simulink model "otonomvehicle"  (R2021b)
settings: Solver=VariableStepAuto  StartTime=0.0  StopTime=50  RelTol=1e-3
libraries: sim3dautolib x3, vrlib x2, simulink x2, sim3dlib x1, mpcadaslib x1, slpidlib x1
settings Model: Creator=serih  LastModifiedBy=serih

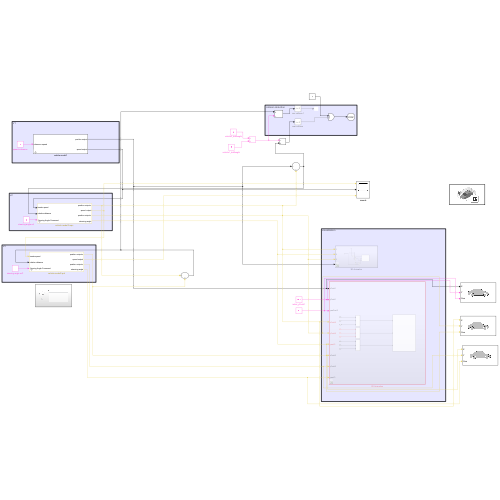
[thumbnail: Simulink's stored preview of the top-level diagram]
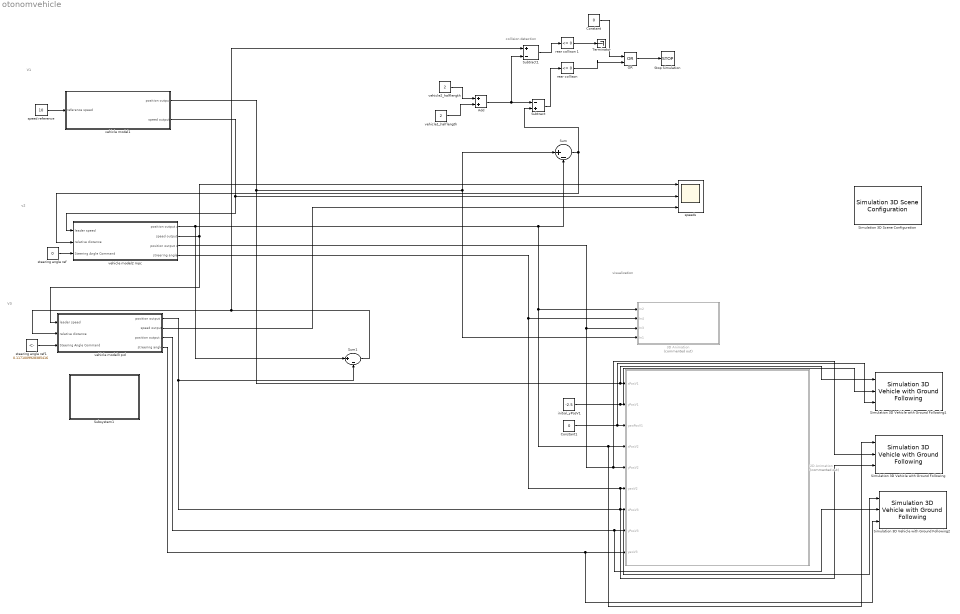
== system otonomvehicle ==
  note: V3
  note: v2
  note: V1
  note: visualization
  note: collision detection
  2D Animation : Subsystem  Commented=on  TreatAsAtomicUnit=on  SystemSampleTime=0.02
  3D Animation : Subsystem  Commented=on
  Add : Sum
  Constant : Constant  Value=0
  Constant1 : Constant  Value=0
  OR : Logic  Operator=OR  IconShape=distinctive  AllPortsSameDT=off  OutDataTypeStr=boolean
  Simulation 3D Scene Configuration : sim3dlib/Simulation 3D Scene Configuration  Priority=0  ProjectFormat_internal=Default Scenes  ProjectFormat=Default Scenes  SceneDesc=Straight road  ProjectName=C:\Program Files\MATLAB\R2021b\toolbox\shared\sim3d_projects\automotive_project\UE4\WindowsNoEditor\VehicleSimulation.exe  ScenePath=/Game/Maps/HwStrght  vehTagList={'Scene Origin';'SimulinkVehicle1';'SimulinkVehicle2';'SimulinkVehicle3'}  vehTag=SimulinkVehicle3  OpVisEn=off  Ts=0.1  EnableWindow=on  EnableWeather=off  SunAltitude=40.0  SunAzimuth=90  clouds=10  wind=1  fog=0  rain=0  sensorTag=MainCamera1  sensorId=1  sensorName=MainCamera1  mountLoc=Origin  offsetFlag=off  tmountOffset=[0, 0, 0]  rmountOffset=[0, 0, 0]  HorizontalResolution=1280  VerticalResolution=720  HorizontalFOV=60  mountPoint=[0 0 0]  mountOrientation=[0 0 0]  aMode=3  ID=1
      link override Simulation 3D Engine: SceneDesc=Straight road  EnableWeather=off  WeatherConfigParas=[40.0,90,10,0,0,1]
      settings: SourceProductBaseCode=AE,DR,UV,VE
  Simulation 3D Vehicle with Ground Following : sim3dautolib/Simulation 3D Vehicle with Ground Following  Priority=-1  PassVehMesh=Sport utility vehicle  PassVehMesh_Internal=Sport utility vehicle  MeshPath=/MathWorksSimulation/Vehicles/Muscle/Meshes/SK_MuscleCar.SK_MuscleCar  TrackWidth=1.9  WheelBase=3  WheelRadius=0.35  VehColor=Green  VehColor_Internal=Green  InitialPos=[20, 0, 0]  InitialRot=[0, 0, 0]  ActorName=SimulinkVehicle1  SampleTime=0.1  ActorType=SimulinkVehicle  ID=1  aMode=3  ActorTag=SimulinkVehicle1  CoordinateScheme=ISO  VehLightsControl=off  HeadlightColor=[ 1, 1, 1 ]  HighBeamIntensity=100000  LowBeamIntensity=60000  HighBeamConeAngle=70  LowBeamConeAngle=70  LeftHeadlightOrientation=[ 0, 0 ]  RightHeadlightOrientation=[ 0, 0 ]  BrakelightIntensity=500  ReverselightIntensity=500  SignallightIntensity=500  SignallightPeriod=1  SignalPulseWidth=50  TransformOutportEnabled=off
      settings: SourceProductBaseCode=AE,DR,UV,VE
  Simulation 3D Vehicle with Ground Following1 : sim3dautolib/Simulation 3D Vehicle with Ground Following  Priority=-1  PassVehMesh=Sedan  PassVehMesh_Internal=Sedan  MeshPath=/MathWorksSimulation/Vehicles/Muscle/Meshes/SK_MuscleCar.SK_MuscleCar  TrackWidth=1.9  WheelBase=3  WheelRadius=0.35  VehColor=Red  VehColor_Internal=Red  InitialPos=[40, 0, 0]  InitialRot=[0, 0, 0]  ActorName=SimulinkVehicle2  SampleTime=0.1  ActorType=SimulinkVehicle  ID=2  aMode=3  ActorTag=SimulinkVehicle2  CoordinateScheme=ISO  VehLightsControl=off  HeadlightColor=[ 1, 1, 1 ]  HighBeamIntensity=100000  LowBeamIntensity=60000  HighBeamConeAngle=70  LowBeamConeAngle=70  LeftHeadlightOrientation=[ 0, 0 ]  RightHeadlightOrientation=[ 0, 0 ]  BrakelightIntensity=500  ReverselightIntensity=500  SignallightIntensity=500  SignallightPeriod=1  SignalPulseWidth=50  TransformOutportEnabled=off
      settings: SourceProductBaseCode=AE,DR,UV,VE
  Simulation 3D Vehicle with Ground Following2 : sim3dautolib/Simulation 3D Vehicle with Ground Following  Priority=-1  PassVehMesh=Hatchback  PassVehMesh_Internal=Hatchback  MeshPath=/MathWorksSimulation/Vehicles/Muscle/Meshes/SK_MuscleCar.SK_MuscleCar  TrackWidth=1.9  WheelBase=3  WheelRadius=0.35  VehColor=Yellow  VehColor_Internal=Yellow  InitialPos=[0, 0, 0]  InitialRot=[0, 0, 0]  ActorName=SimulinkVehicle3  SampleTime=0.1  ActorType=SimulinkVehicle  ID=3  aMode=3  ActorTag=SimulinkVehicle3  CoordinateScheme=ISO  VehLightsControl=off  HeadlightColor=[ 1, 1, 1 ]  HighBeamIntensity=100000  LowBeamIntensity=60000  HighBeamConeAngle=70  LowBeamConeAngle=70  LeftHeadlightOrientation=[ 0, 0 ]  RightHeadlightOrientation=[ 0, 0 ]  BrakelightIntensity=500  ReverselightIntensity=500  SignallightIntensity=500  SignallightPeriod=1  SignalPulseWidth=50  TransformOutportEnabled=off
      settings: SourceProductBaseCode=AE,DR,UV,VE
  Stop Simulation : Stop
  Subsystem1 : Subsystem
  Subtract : Sum  Inputs=-+
  Subtract1 : Sum  Inputs=+-
  Sum : Sum  Inputs=|+-
  Sum1 : Sum  Inputs=|+-
  Terminator : Terminator
  initial_yPosV1 : Constant  Value=-2.5
  "rear collison " : simulink/Logic and Bit Operations/Compare To Constant  relop=<=  const=0  OutDataTypeStr=boolean
  rear collison 1 : simulink/Logic and Bit Operations/Compare To Constant  relop=<=  const=0  OutDataTypeStr=boolean
  speed reference : Constant  Value=10
  speeds : Scope  NumInputPorts=3
  steering angle ref : Constant  Value=0  VectorParams1D=off
  steering angle ref1 : Constant  Value=0.1171009928385416  VectorParams1D=off
  vehicle model1 : Subsystem  mask{pos=30, speed=20}
      mask prompts: pos "initial position"; speed "initial speed"
      mask TypeOptions pos: initial position/Value
      mask TypeOptions speed: initial speed/Value
  "vehicle model2 mpc " : Subsystem  mask{pos=20, speed=15}
      mask prompts: pos "initial position"; speed "initial speed"
      mask TypeOptions pos: initial position z/Value
      mask TypeOptions speed: initial speed/Value
  vehicle model3 pıd : Subsystem  mask{pos=0, speed=20}
      mask prompts: pos "initial position"; speed "initial speed"
      mask TypeOptions pos: initial position z/Value
      mask TypeOptions speed: initial speed/Value
  vehicle1_halflength : Constant  Value=2
  vehicle2_halflength : Constant  Value=2
  wires:
  speed reference/1 -> vehicle model1/1(reference speed)
  vehicle model1/1(position output) -> Simulation 3D Vehicle with Ground Following1/1, 2D Animation/1(xPosV1), 3D Animation/4(In1), Sum/1
  "vehicle model2 mpc "/1(position output z) -> Sum1/1, Sum/2, 3D Animation/1(In2), Simulation 3D Vehicle with Ground Following/1, 2D Animation/4(xPosV2)
  vehicle model1/2(speed output) -> speeds/2, "vehicle model2 mpc "/1(leader speed)
  Sum/1 -> Subtract/2, "vehicle model2 mpc "/2(relative distance)
  steering angle ref/1 -> "vehicle model2 mpc "/3(Steering Angle Command)
  "vehicle model2 mpc "/3(position output x) -> Simulation 3D Vehicle with Ground Following/2, 2D Animation/5(yPosV2), 3D Animation/3(In3)
  "vehicle model2 mpc "/4(streering angle) -> Simulation 3D Vehicle with Ground Following/3, 2D Animation/6(yawV2), 3D Animation/2(In4)
  Constant1/1 -> 2D Animation/3(yawPosV1), Simulation 3D Vehicle with Ground Following1/3
  initial_yPosV1/1 -> Simulation 3D Vehicle with Ground Following1/2, 2D Animation/2(yPosV1)
  vehicle2_halflength/1 -> Add/1
  vehicle1_halflength/1 -> Add/2
  Add/1 -> Subtract1/2, Subtract/1
  Subtract/1 -> "rear collison "/1
  Subtract1/1 -> rear collison 1/1
  OR/1 -> Stop Simulation/1
  "rear collison "/1 -> OR/2
  "vehicle model2 mpc "/2(speed output) -> vehicle model3 pıd/1(leader speed), speeds/1
  vehicle model3 pıd/1(position output z) -> Simulation 3D Vehicle with Ground Following2/1, 2D Animation/7(xPosV3), Sum1/2
  Sum1/1 -> vehicle model3 pıd/2(relative distance), Subtract1/1
  steering angle ref1/1 -> vehicle model3 pıd/3(Steering Angle Command)
  vehicle model3 pıd/2(speed output) -> speeds/3
  vehicle model3 pıd/4(streering angle) -> Simulation 3D Vehicle with Ground Following2/3, 2D Animation/9(yawV3)
  vehicle model3 pıd/3(position output x) -> 2D Animation/8(yPosV3), Simulation 3D Vehicle with Ground Following2/2
  rear collison 1/1 -> Terminator/1
  Constant/1 -> OR/1

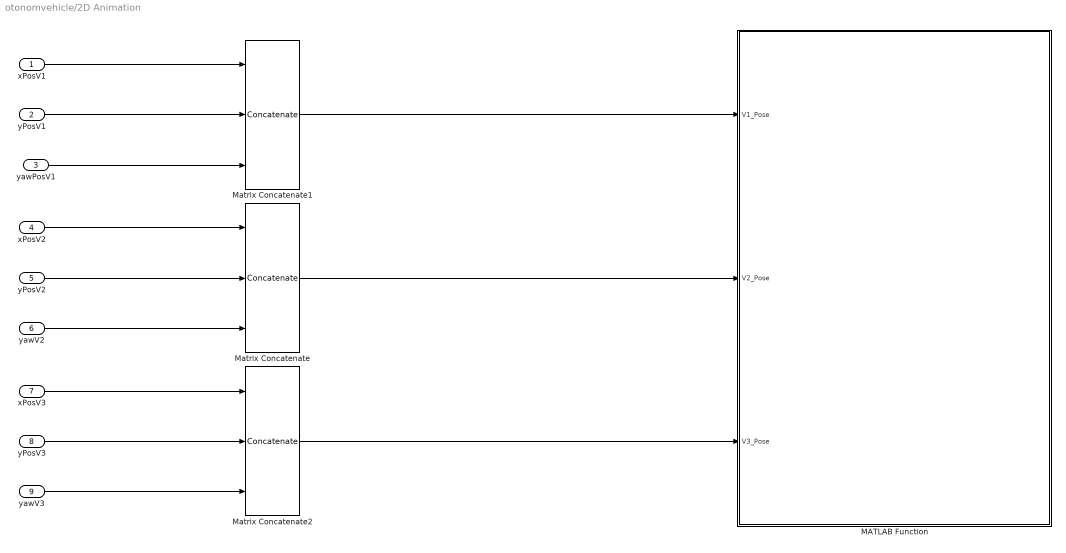
== system otonomvehicle/2D Animation ==
  xPosV1 : Inport
  yPosV1 : Inport  Port=2
  yawPosV1 : Inport  Port=3
  xPosV2 : Inport  Port=4
  yPosV2 : Inport  Port=5
  yawV2 : Inport  Port=6
  xPosV3 : Inport  Port=7
  yPosV3 : Inport  Port=8
  yawV3 : Inport  Port=9
  MATLAB Function : MATLAB Function  TreatAsAtomicUnit=on
      mask init:
      | close all;
      | figure('units','normalized','outerposition',[0 0 1 1 ]);
      | grid on
      | axis equal
      | hold on
  Matrix Concatenate : Concatenate  NumInputs=3  ConcatenateDimension=2
  Matrix Concatenate1 : Concatenate  NumInputs=3  ConcatenateDimension=2
  Matrix Concatenate2 : Concatenate  NumInputs=3  ConcatenateDimension=2
  wires:
  xPosV2/1 -> Matrix Concatenate/1
  yPosV2/1 -> Matrix Concatenate/2
  yawV2/1 -> Matrix Concatenate/3
  Matrix Concatenate/1 -> MATLAB Function/2(V2_Pose)
  Matrix Concatenate1/1 -> MATLAB Function/1(V1_Pose)
  xPosV1/1 -> Matrix Concatenate1/1
  yPosV1/1 -> Matrix Concatenate1/2
  yawPosV1/1 -> Matrix Concatenate1/3
  xPosV3/1 -> Matrix Concatenate2/1
  yPosV3/1 -> Matrix Concatenate2/2
  yawV3/1 -> Matrix Concatenate2/3
  Matrix Concatenate2/1 -> MATLAB Function/3(V3_Pose)

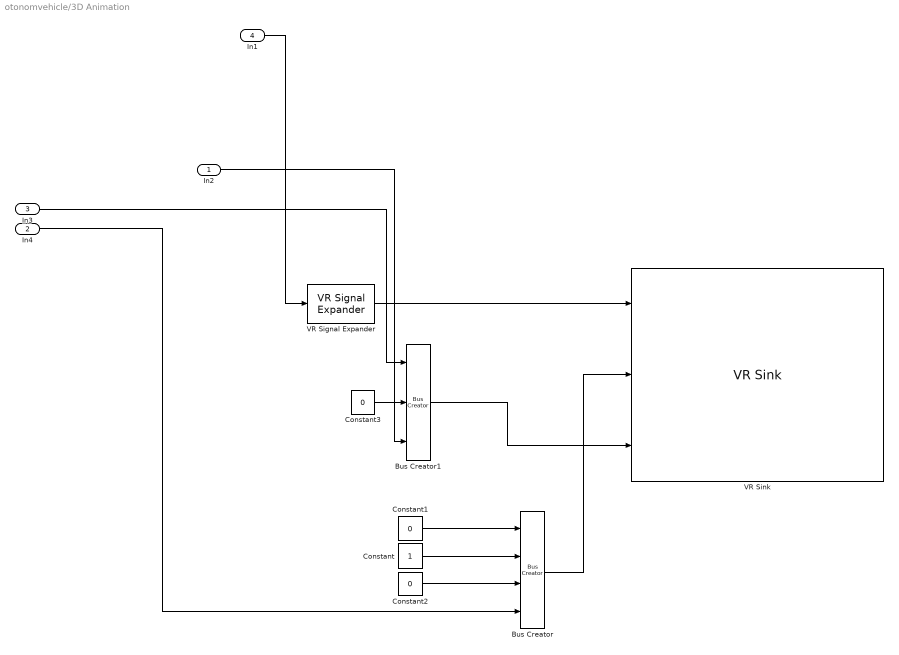
== system otonomvehicle/3D Animation ==
  In2 : Inport
  In4 : Inport  Port=2
  In3 : Inport  Port=3
  In1 : Inport  Port=4
  Bus Creator : BusCreator  Inputs=4
  Bus Creator1 : BusCreator  Inputs=3
  Constant : Constant
  Constant1 : Constant  Value=0
  Constant2 : Constant  Value=0
  Constant3 : Constant  Value=0
  VR Signal Expander : vrlib/VR Signal Expander  outwidth=3  outidx=[3]
  VR Sink : vrlib/VR Sink  InstantiateOnLoad=on  SampleTime=0.02  ViewEnable=on  RemoteChange=off  RemoteView=off  FieldsWritten=Car_Red.translation.3.1.1.double#Car_Blue.rotation.4.1.1.double#Car_Blue.translation.3.1.1.double  WorldFileName=OneDrive\Masaüstü\PlatoonWorld.WRL  AutoView=off  VideoDimensions=[]  AllowVariableSize=off
  wires:
  Constant1/1 -> Bus Creator/1
  VR Signal Expander/1 -> VR Sink/1
  In1/1 -> VR Signal Expander/1
  Constant2/1 -> Bus Creator/3
  Bus Creator/1 -> VR Sink/2
  Constant3/1 -> Bus Creator1/2
  Constant/1 -> Bus Creator/2
  Bus Creator1/1 -> VR Sink/3
  In3/1 -> Bus Creator1/1
  In4/1 -> Bus Creator/4
  In2/1 -> Bus Creator1/3

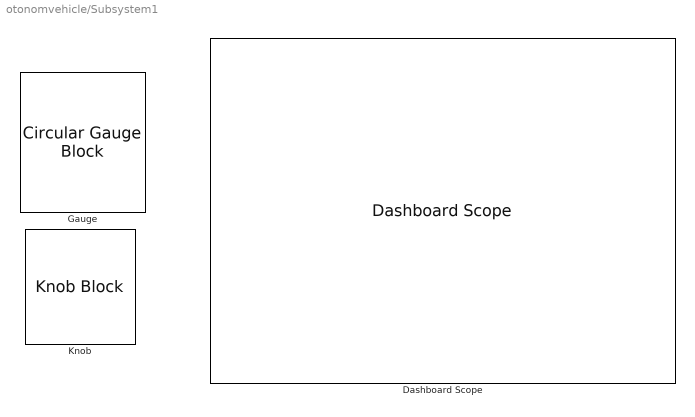
== system otonomvehicle/Subsystem1 ==
  Dashboard Scope : DashboardScope
  Gauge : CircularGaugeBlock
  Knob : KnobBlock  ScaleMin=-0.2  ScaleMax=0.2

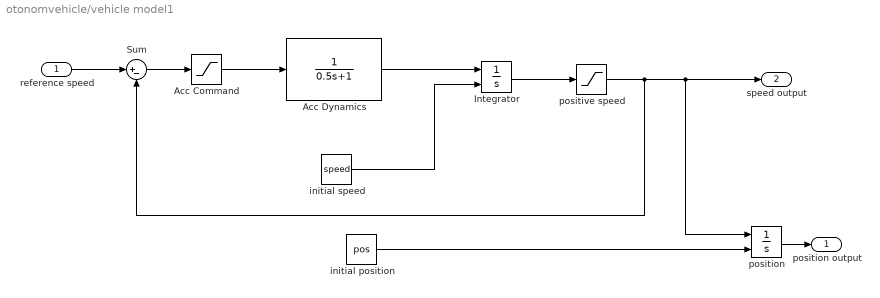
== system otonomvehicle/vehicle model1 ==
  reference speed : Inport
  Acc Command : Saturate  UpperLimit=2  LowerLimit=-3
  Acc Dynamics : TransferFcn  Denominator=[0.5 1]
  Integrator : Integrator  InitialConditionSource=external
  Sum : Sum  Inputs=|+-
  initial position : Constant  Value=pos
  initial speed : Constant  Value=speed
  position : Integrator  InitialConditionSource=external
  positive speed : Saturate  UpperLimit=inf  LowerLimit=0
  position output : Outport
  speed output : Outport  Port=2
  wires:
  Sum/1 -> Acc Command/1
  positive speed/1 -> speed output/1, position/1, Sum/2
  initial speed/1 -> Integrator/2
  initial position/1 -> position/2
  Acc Command/1 -> Acc Dynamics/1
  reference speed/1 -> Sum/1
  Acc Dynamics/1 -> Integrator/1
  Integrator/1 -> positive speed/1
  position/1 -> position output/1

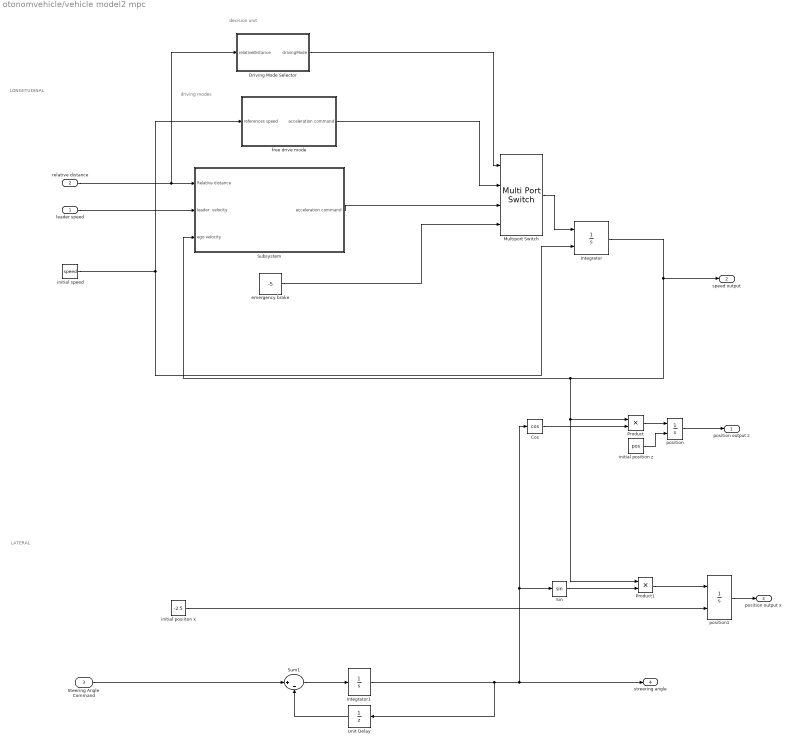
== system otonomvehicle/vehicle model2 mpc  ==
  note: decision unit
  note: driving modes
  note: LATERAL
  note: LONGIITUDINAL
  leader speed : Inport
  relative distance : Inport  Port=2
  Steering Angle Command : Inport  Port=3
  Cos : Trigonometry  Operator=cos
  Driving Mode Selector : Stateflow chart  TreatAsAtomicUnit=on
  Integrator : Integrator  InitialConditionSource=external  LimitOutput=on  LowerSaturationLimit=0
  Integrator1 : Integrator
  Multiport Switch : MultiPortSwitch
  Product : Product
  Product1 : Product
  Sin : Trigonometry
  Subsystem : Subsystem
  Sum1 : Sum  Inputs=|+-
  Unit Delay : UnitDelay  SampleTime=-1  HasFrameUpgradeWarning=on
  emergency brake : Constant  Value=-5
  free drive mode : Subsystem
  initial posiiton x : Constant  Value=-2.5
  initial position z : Constant  Value=pos
  initial speed : Constant  Value=speed
  position : Integrator  InitialConditionSource=external
  position1 : Integrator  InitialConditionSource=external
  position output z : Outport
  speed output : Outport  Port=2
  position output x : Outport  Port=3
  streering angle : Outport  Port=4
  wires:
  initial speed/1 -> Integrator/2, free drive mode/1(references speed)
  initial position z/1 -> position/2
  position/1 -> position output z/1
  Integrator/1 -> Subsystem/3("ego velocity "), Product1/1, Product/1, speed output/1
  Steering Angle Command/1 -> Sum1/1
  Sum1/1 -> Integrator1/1
  Integrator1/1 -> Unit Delay/1, streering angle/1, Cos/1, Sin/1
  Unit Delay/1 -> Sum1/2
  initial posiiton x/1 -> position1/2
  Cos/1 -> Product/2
  Product/1 -> position/1
  Sin/1 -> Product1/2
  Product1/1 -> position1/1
  position1/1 -> position output x/1
  relative distance/1 -> Driving Mode Selector/1(relativeDistance), Subsystem/1(Relative distance)
  leader speed/1 -> Subsystem/2("leader  velocity ")
  Multiport Switch/1 -> Integrator/1
  emergency brake/1 -> Multiport Switch/4
  Subsystem/1("acceleration command ") -> Multiport Switch/3
  free drive mode/1(acceleration command) -> Multiport Switch/2
  Driving Mode Selector/1(drivingMode) -> Multiport Switch/1

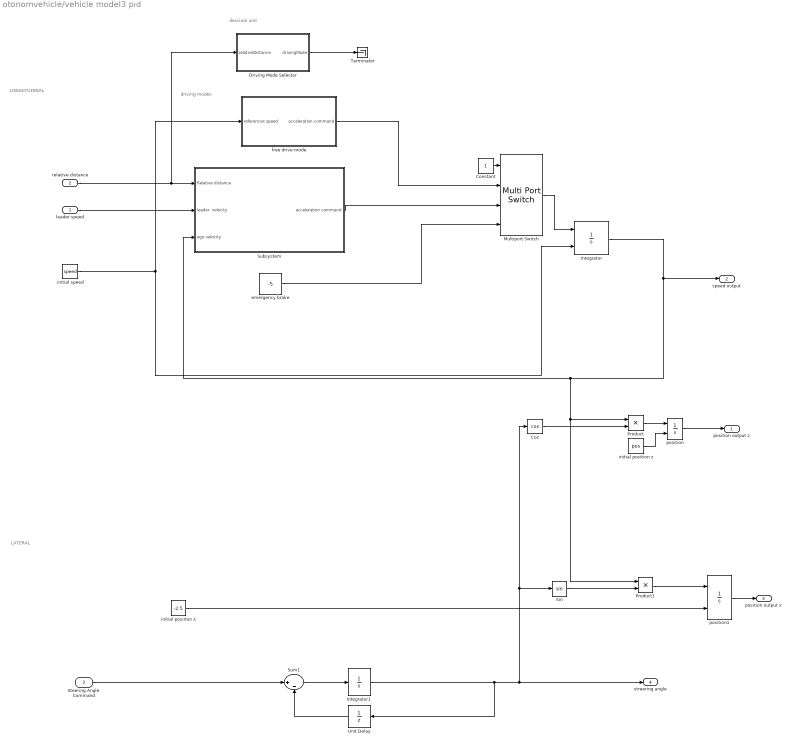
== system otonomvehicle/vehicle model3 pıd ==
  note: decision unit
  note: driving modes
  note: LATERAL
  note: LONGIITUDINAL
  leader speed : Inport
  relative distance : Inport  Port=2
  Steering Angle Command : Inport  Port=3
  Constant : Constant
  Cos : Trigonometry  Operator=cos
  Driving Mode Selector : Stateflow chart  TreatAsAtomicUnit=on
  Integrator : Integrator  InitialConditionSource=external  LimitOutput=on
  Integrator1 : Integrator
  Multiport Switch : MultiPortSwitch
  Product : Product
  Product1 : Product
  Sin : Trigonometry
  Subsystem : Subsystem
  Sum1 : Sum  Inputs=|+-
  Terminator : Terminator
  Unit Delay : UnitDelay  SampleTime=-1  HasFrameUpgradeWarning=on
  emergency brake : Constant  Value=-5
  free drive mode : Subsystem
  initial posiiton x : Constant  Value=-2.5
  initial position z : Constant  Value=pos
  initial speed : Constant  Value=speed
  position : Integrator  InitialConditionSource=external
  position1 : Integrator  InitialConditionSource=external
  position output z : Outport
  speed output : Outport  Port=2
  position output x : Outport  Port=3
  streering angle : Outport  Port=4
  wires:
  initial speed/1 -> Integrator/2, free drive mode/1(references speed)
  initial position z/1 -> position/2
  position/1 -> position output z/1
  Integrator/1 -> Subsystem/3("ego velocity "), Product1/1, Product/1, speed output/1
  Steering Angle Command/1 -> Sum1/1
  Sum1/1 -> Integrator1/1
  Integrator1/1 -> Unit Delay/1, streering angle/1, Cos/1, Sin/1
  Unit Delay/1 -> Sum1/2
  initial posiiton x/1 -> position1/2
  Cos/1 -> Product/2
  Product/1 -> position/1
  Sin/1 -> Product1/2
  Product1/1 -> position1/1
  position1/1 -> position output x/1
  relative distance/1 -> Driving Mode Selector/1(relativeDistance), Subsystem/1(Relative distance)
  leader speed/1 -> Subsystem/2("leader  velocity ")
  Multiport Switch/1 -> Integrator/1
  emergency brake/1 -> Multiport Switch/4
  Subsystem/1("acceleration command ") -> Multiport Switch/3
  free drive mode/1(acceleration command) -> Multiport Switch/2
  Driving Mode Selector/1(drivingMode) -> Terminator/1
  Constant/1 -> Multiport Switch/1

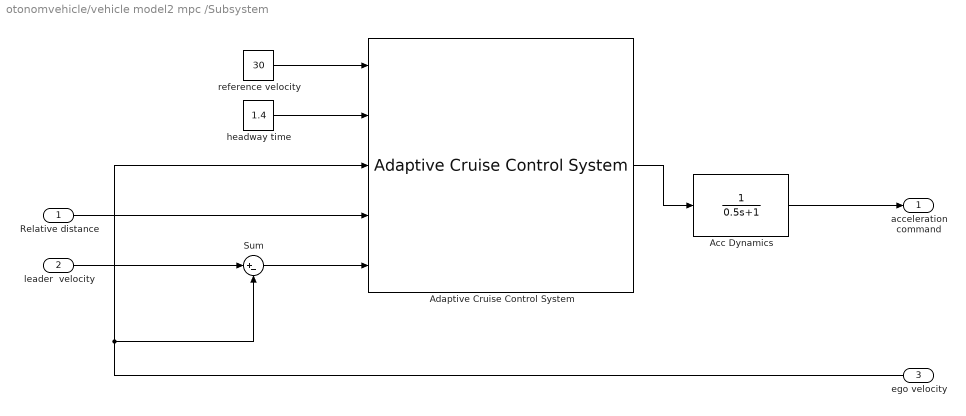
== system otonomvehicle/vehicle model2 mpc /Subsystem ==
  Relative distance : Inport
  "leader  velocity " : Inport  Port=2
  "ego velocity " : Inport  Port=3
  Acc Dynamics : TransferFcn  Denominator=[0.5 1]
  Adaptive Cruise Control System : mpcadaslib/Adaptive Cruise Control System  EgoModel=tf(1,[0.5,1,0])  InitialEgoVelocity=30  DefaultSpacing=10  MaxVelocity=50  MinAcceleration=-3  amin_ext=off  MaxAcceleration=2  amax_ext=off  Ts=0.5  PredictionHorizon=200  ControllerBehavior=0.590  suboptimal=off  maxiter=10  datatypeopt=double  optmode=off  trackmode=off
  Sum : Sum  Inputs=|+-
  headway time : Constant  Value=1.4
  reference velocity : Constant  Value=30
  "acceleration command " : Outport
  wires:
  Sum/1 -> Adaptive Cruise Control System/5
  headway time/1 -> Adaptive Cruise Control System/2
  Adaptive Cruise Control System/1 -> Acc Dynamics/1
  Acc Dynamics/1 -> "acceleration command "/1
  "leader  velocity "/1 -> Sum/1
  "ego velocity "/1 -> Sum/2, Adaptive Cruise Control System/3
  reference velocity/1 -> Adaptive Cruise Control System/1
  Relative distance/1 -> Adaptive Cruise Control System/4

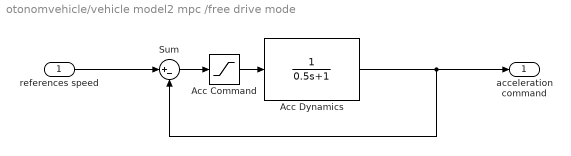
== system otonomvehicle/vehicle model2 mpc /free drive mode ==
  references speed : Inport
  Acc Command : Saturate  UpperLimit=2  LowerLimit=-3
  Acc Dynamics : TransferFcn  Denominator=[0.5 1]
  Sum : Sum  Inputs=|+-
  acceleration command : Outport
  wires:
  Sum/1 -> Acc Command/1
  references speed/1 -> Sum/1
  Acc Dynamics/1 -> Sum/2, acceleration command/1
  Acc Command/1 -> Acc Dynamics/1

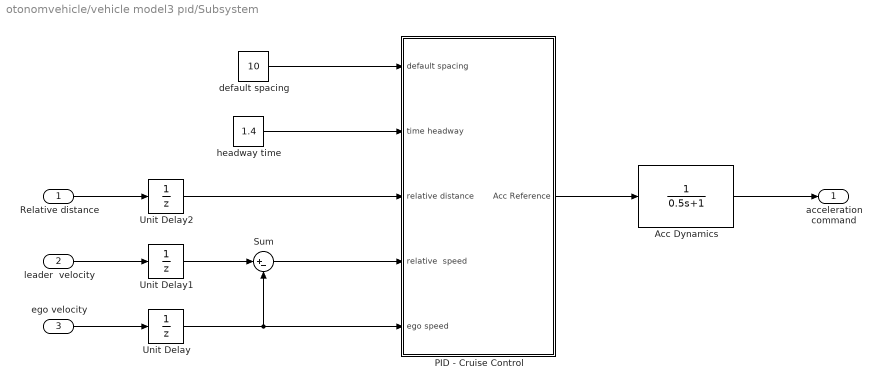
== system otonomvehicle/vehicle model3 pıd/Subsystem ==
  Relative distance : Inport
  "leader  velocity " : Inport  Port=2
  "ego velocity " : Inport  Port=3
  " default spacing" : Constant  Value=10
  Acc Dynamics : TransferFcn  Denominator=[0.5 1]
  PID - Cruise Control : Subsystem
  Sum : Sum  Inputs=|+-
  Unit Delay : UnitDelay  SampleTime=-1  HasFrameUpgradeWarning=on
  Unit Delay1 : UnitDelay  SampleTime=-1  HasFrameUpgradeWarning=on
  Unit Delay2 : UnitDelay  SampleTime=-1  HasFrameUpgradeWarning=on
  headway time : Constant  Value=1.4
  "acceleration command " : Outport
  wires:
  Sum/1 -> PID - Cruise Control/4(relative  speed)
  headway time/1 -> PID - Cruise Control/2(time headway)
  PID - Cruise Control/1(Acc Reference) -> Acc Dynamics/1
  Acc Dynamics/1 -> "acceleration command "/1
  Relative distance/1 -> Unit Delay2/1
  " default spacing"/1 -> PID - Cruise Control/1(default spacing)
  "ego velocity "/1 -> Unit Delay/1
  Unit Delay/1 -> Sum/2, PID - Cruise Control/5(ego speed)
  "leader  velocity "/1 -> Unit Delay1/1
  Unit Delay1/1 -> Sum/1
  Unit Delay2/1 -> PID - Cruise Control/3(relative distance)

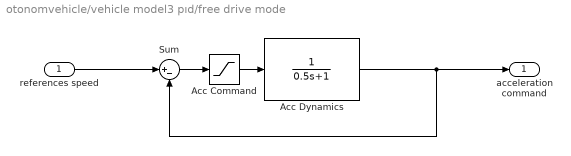
== system otonomvehicle/vehicle model3 pıd/free drive mode ==
  references speed : Inport
  Acc Command : Saturate  UpperLimit=2  LowerLimit=-3
  Acc Dynamics : TransferFcn  Denominator=[0.5 1]
  Sum : Sum  Inputs=|+-
  acceleration command : Outport
  wires:
  Sum/1 -> Acc Command/1
  references speed/1 -> Sum/1
  Acc Dynamics/1 -> Sum/2, acceleration command/1
  Acc Command/1 -> Acc Dynamics/1

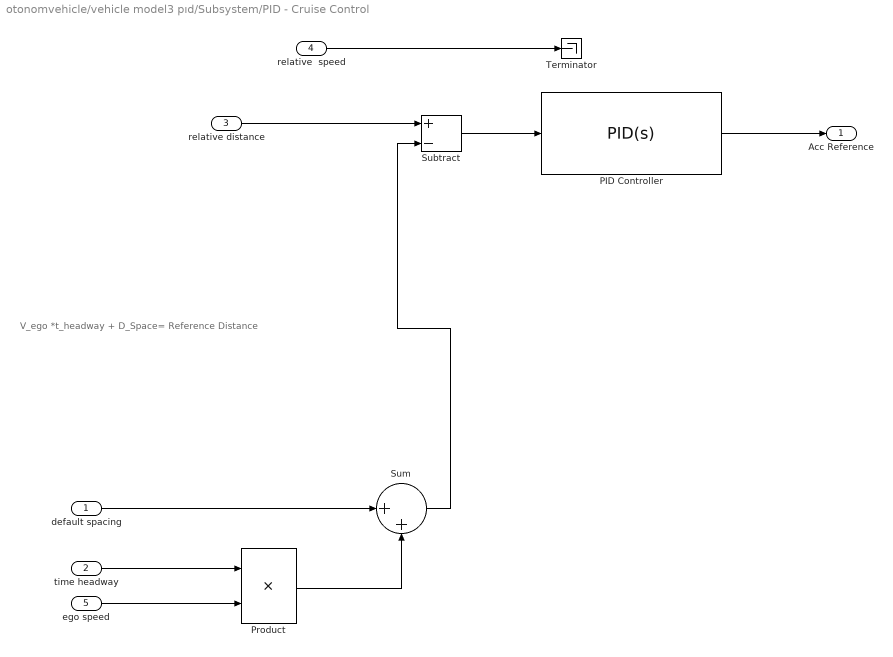
== system otonomvehicle/vehicle model3 pıd/Subsystem/PID - Cruise Control ==
  note: V_ego *t_headway + D_Space= Reference Distance
  default spacing : Inport
  time headway : Inport  Port=2
  relative distance : Inport  Port=3
  relative  speed : Inport  Port=4
  ego speed : Inport  Port=5
  PID Controller : slpidlib/PID Controller  Controller=PID  Form=Parallel  TimeDomain=Continuous-time  UseExternalTs=off  SampleTime=-1  IntegratorMethod=Forward Euler  FilterMethod=Forward Euler  ControllerParametersSource=internal  P=2  I=0.04  D=2.1  UseFilter=on  N=230  TunerSelectOption=Transfer Function Based (PID Tuner App)  InitialConditionSource=internal  InitialConditionForIntegrator=0  InitialConditionForFilter=0  DifferentiatorICPrevScaledInput=0  ExternalReset=none  TrackingMode=off  Kt=1  LimitOutput=on  SatLimitsSource=internal  UpperSaturationLimit=2  LowerSaturationLimit=-3  LinearizeAsGain=on  AntiWindupMode=clamping  Kb=1  POutMin=[]  POutMax=[]  IOutMin=[]  IOutMax=[]  DOutMin=[]  DOutMax=[]  NOutMin=[]  NOutMax=[]  SumOutMin=[]  SumOutMax=[]  SaturationOutMin=[]  SaturationOutMax=[]  PParamMin=[]  PParamMax=[]  IParamMin=[]  IParamMax=[]  DParamMin=[]  DParamMax=[]  NParamMin=[]  NParamMax=[]  KbParamMin=[]  KbParamMax=[]  KtParamMin=[]  KtParamMax=[]  KbOutMin=[]  KbOutMax=[]  KtOutMin=[]  KtOutMax=[]  IntegratorOutMin=[]  IntegratorOutMax=[]  FilterOutMin=[]  FilterOutMax=[]  SumI1OutMin=[]  SumI1OutMax=[]  SumI2OutMin=[]  SumI2OutMax=[]  SumI3OutMin=[]  SumI3OutMax=[]  SumI4OutMin=[]  SumI4OutMax=[]  SumDOutMin=[]  SumDOutMax=[]  DifferentiatorOutMin=[]  DifferentiatorOutMax=[]  FilterDiffOutCoefMin=[]  FilterDiffOutCoefMax=[]  ReciprocalOutMin=[]  ReciprocalOutMax=[]  SumDenOutMin=[]  SumDenOutMax=[]  SumNumOutMin=[]  SumNumOutMax=[]  DivideOutMin=[]  DivideOutMax=[]  UdiffTsProdOutMin=[]  UdiffTsProdOutMax=[]  NTsProdOutMin=[]  NTsProdOutMax=[]  UintegralTsProdOutMin=[]  UintegralTsProdOutMax=[]  UngainTsProdOutMin=[]  UngainTsProdOutMax=[]  IntegratorContinuousStateAttributes=''  IntegratorStateMustResolveToSignalObject=off  IntegratorRTWStateStorageClass=Auto  FilterContinuousStateAttributes=''  FilterStateMustResolveToSignalObject=off  FilterRTWStateStorageClass=Auto  ParallelPVariant=InternalParameters  IdealPVariant=Disabled  IVariant=InternalParameters  DVariant=InternalParameters  IntegratorVariant=Continuous  SatVariant=Enabled  AWVariant=ContClampingParallel  PCopyVariant=Disabled  TRVariant=Disabled  FdbkBlocksVariant=Forward  IdealPFdbkVariant=Disabled  SatFdbkVariant=Disabled  DerivativeFilterVariant=ContFilter  NVariant=InternalParameters  NCopyVariant=Disabled  FilterICVariant=InternalICsFilter  IntegratorICVariant=InternalICs  ExternalResetVariant=Disabled  TRSumVariant=Passthrough  SumFdbkVariant=Disabled  SumVariant=Sum_PID  TsampFilterVariant=InternalTs  TsampNgainVariant=Passthrough  TsampIntegralVariant=Passthrough  ExternalSaturationOutDataTypeStr=Inherit: Same as second input
  Product : Product
  Subtract : Sum  Inputs=+-
  Sum : Sum  Inputs=|++
  Terminator : Terminator
  Acc Reference : Outport
  wires:
  ego speed/1 -> Product/2
  time headway/1 -> Product/1
  Product/1 -> Sum/2
  default spacing/1 -> Sum/1
  Sum/1 -> Subtract/2
  relative distance/1 -> Subtract/1
  Subtract/1 -> PID Controller/1
  PID Controller/1 -> Acc Reference/1
  relative  speed/1 -> Terminator/1

== stateflow chart otonomvehicle/vehicle model3 pıd/Driving Mode Selector ==
  state FreeDrive
    entry:
    drivingMode=1;
  state VehicleFollowing
    entry:
    drivingMode=2;
  state EmergencyBrake
    entry:
    drivingMode=3;
  (default) -> FreeDrive
  VehicleFollowing -> FreeDrive [order 1] : [relativeDistance>50]
  FreeDrive -> VehicleFollowing : [relativeDistance <=40]
  EmergencyBrake -> FreeDrive [order 1] : [relativeDistance<=10]
  VehicleFollowing -> EmergencyBrake [order 2] : [relativeDistance<=10]
  EmergencyBrake -> VehicleFollowing [order 2] : [relativeDistance>15]
  data: relativeDistance input; drivingMode output

== matlab function otonomvehicle/2D Animation/MATLAB Function ==
  data: V1_Pose input; V2_Pose input; V3_Pose input
function plotVehicle(V1_Pose,V2_Pose,V3_Pose)
%%clear previous vehicle 
cla
%% vehicle-1 pose
x1=V1_Pose(1);
y1=V1_Pose(2);
yaw1=V1_Pose(3);
centerP=[x1;y1];

V1_HalfLength=2; %length 4 meters
V1_HalfWidth=1; %width 2 meters 

%creating a rectangle
p1=[V1_HalfLength; V1_HalfWidth];
p2=[V1_HalfLength; -V1_HalfWidth];
p3=[-V1_HalfLength; -V1_HalfWidth];
p4=[-V1_HalfLength; V1_HalfWidth];

%rotation matrix
Rmatrix=[cos(yaw1) -sin(yaw1);  sin(yaw1) cos(yaw1)];

%rotated points
p1r= centerP + Rmatrix*p1;
p2r= centerP + Rmatrix*p2;
p3r= centerP + Rmatrix*p3;
p4r= centerP + Rmatrix*p4;

%connecting points
Hitbox_V1= [p1r p2r p3r p4r p1r];

cornersV1_x= transpose(Hitbox_V1(1,:));
cornersV1_y= transpose(Hitbox_V1(2,:));


%% vehicle-2 pose
x2=V2_Pose(1);
y2=V2_Pose(2);
yaw2=V2_Pose(3);

centerP=[x2;y2];

V2_HalfLength=2; %length 4 meters
V2_HalfWidth=1; %width 2 meters 

%creating a rectangle
p1=[V2_HalfLength; V2_HalfWidth];
p2=[V2_HalfLength; -V2_HalfWidth];
p3=[-V2_HalfLength; -V2_HalfWidth];
p4=[-V2_HalfLength; V2_HalfWidth];

%rotation matrix
Rmatrix=[cos(yaw2) -sin(yaw2);  sin(yaw2) cos(yaw2)];

%rotated points
p1r= centerP + Rmatrix*p1;
p2r= centerP + Rmatrix*p2;
p3r= centerP + Rmatrix*p3;
p4r= centerP + Rmatrix*p4;

%connecting points
Hitbox_V2= [p1r p2r p3r p4r p1r];

cornersV2_x= transpose(Hitbox_V2(1,:));
cornersV2_y= transpose(Hitbox_V2(2,:));

%% vehicle-3 pose
x3=V3_Pose(1);
y3=V3_Pose(2);
yaw3=V3_Pose(3);

centerP=[x3;y3];

V3_HalfLength=2; %length 4 meters
V3_HalfWidth=1; %width 2 meters 

%creating a rectangle
p1=[V3_HalfLength; V3_HalfWidth];
p2=[V3_HalfLength; -V3_HalfWidth];
p3=[-V3_HalfLength; -V3_HalfWidth];
p4=[-V3_HalfLength; V3_HalfWidth];

%rotation matrix
Rmatrix=[cos(yaw3) -sin(yaw3);  sin(yaw3) cos(yaw3)];

%rotated points
p1r= centerP + Rmatrix*p1;
p2r= centerP + Rmatrix*p2;
p3r= centerP + Rmatrix*p3;
p4r= centerP + Rmatrix*p4;

%connecting points
Hitbox_V3= [p1r p2r p3r p4r p1r];

cornersV3_x= transpose(Hitbox_V3(1,:));
cornersV3_y= transpose(Hitbox_V3(2,:));

%%plot vehicles
plot(cornersV1_x,cornersV1_y,'g'); %vehicle 1 rectangle
plot(x1,y1,'o'); %vehicle center

plot(cornersV2_x,cornersV2_y,'r'); %vehicle 2 rectangle
plot(x2,y2,'*'); %vehicle center

plot(cornersV3_x,cornersV3_y,'b'); %vehicle 3 rectangle
plot(x3,y3,'x'); %vehicle center

upperLine = plot([0 1000],[5 5],'Color','blue');
midLine = plot([0 1000],[0 0],'--','Color','blue');
lowerLine = plot([0 1000],[-5 -5],'Color','blue');

%adjust axis
axis([x3-40 x3+40 y3-20 y3+20]); % camera following V2 as ego vehicle

== stateflow chart otonomvehicle/vehicle model2 mpc /Driving Mode Selector ==
  state FreeDrive
    entry:
    drivingMode=1;
  state VehicleFollowing
    entry:
    drivingMode=2;
  state EmergencyBrake
    entry:
    drivingMode=3;
  (default) -> FreeDrive
  VehicleFollowing -> FreeDrive [order 1] : [relativeDistance>50]
  FreeDrive -> VehicleFollowing : [relativeDistance <=40]
  EmergencyBrake -> FreeDrive [order 1] : [relativeDistance<=10]
  VehicleFollowing -> EmergencyBrake [order 2] : [relativeDistance<=10]
  EmergencyBrake -> VehicleFollowing [order 2] : [relativeDistance>15]
  data: relativeDistance input; drivingMode output
